simulink model "protocol_nanhang"  (R2023a)
settings: Solver=ode5  StartTime=0.0  StopTime=inf  FixedStep=0.001  RelTol=1e-3
undefined symbols (not defined in the file or in its folder): LF
libraries: instrumentseriallib x6, sldrtlib x1
settings Model: Creator=DELL  LastModifiedBy=DELL
settings HardwareCC: ProdBitPerLong=64  ProdHWDeviceType=Intel->x86-64 (Linux 64)
settings ModelReferenceCC: EnableRefExpFcnMdlSchedulingChecks=on
settings RTWCC: Description=Simulink Desktop Real-Time  SystemTargetFile=sldrt.tlc  TemplateMakefile=sldrt.tmf  RTWCompilerOptimization=on
settings CodeAppCC: MaxIdLength=95
settings SimulinkDesktopRealTimeCC: TargetLibSuffix=_sldrt.a  TargetPreCompLibLocation=C:\Program Files\MATLAB\R2023a\toolbox\sldrt\lib\win64

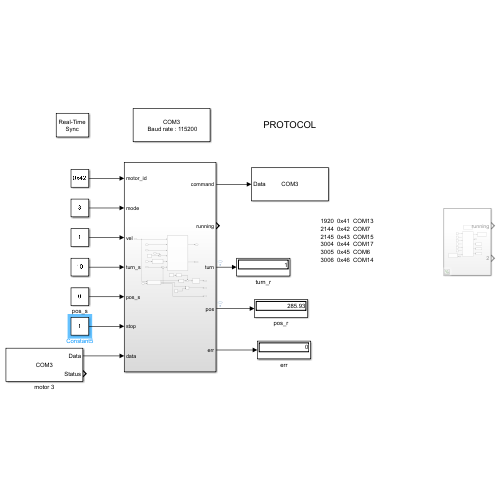
[thumbnail: Simulink's stored preview of the top-level diagram]
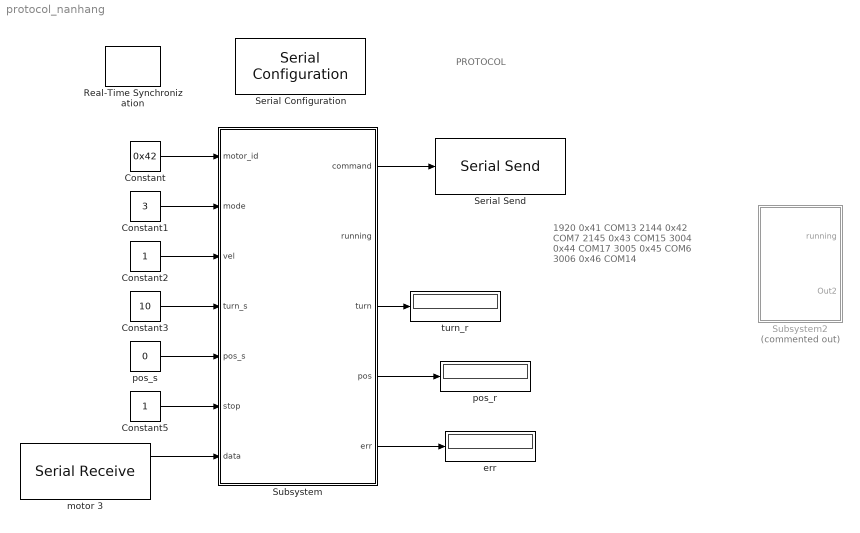
== system protocol_nanhang ==
  note: PROTOCOL
  note: 1920  0x41  COM13
      | 2144  0x42  COM7
      | 2145  0x43  COM15
      | 3004  0x44  COM17
      | 3005  0x45  COM6
      | 3006  0x46  COM14
  Constant : Constant  Value=0x42
  Constant1 : Constant  Value=3
  Constant2 : Constant
  Constant3 : Constant  Value=10
  Constant5 : Constant
  Real-Time Synchronization : sldrtlib/Real-Time Synchronization  SampleTime=0.1  MaxMissedTicks=10  ShowMissedTicks=off  YieldWhenWaiting=off
  Serial Configuration : instrumentseriallib/Serial Configuration  Priority=-200000  PortSel=COM3  Port=COM3  ComPort=COM3  BaudRate=115200  DataBits=8  Parity=none  StopBits=1  ByteOrder=little-endian  FlowControl=none  Timeout=10  SimulateUsing=Interpreted execution  BlockInModel=on  aMode=1
  Serial Send : instrumentseriallib/Serial Send  Priority=1  PortSel=COM3  Port=COM3  ComPort=COM3  Header=[]  Terminator=<none>  CustomTerminator=[]  EnableBlockingMode=off  SimulateUsing=Interpreted execution  BlockInModel=on  aMode=1
  Subsystem : Subsystem
  Subsystem2 : Subsystem  Commented=on
  err : Display
  motor 3 : instrumentseriallib/Serial Receive  Priority=1  PortSel=COM3  Port=COM3  ComPort=COM3  DataType=uint8  SaveDataType=uint8  ToggleHeader=off  Header=[]  ToggleTerminator=on  Terminator=LF ('\n')  CustomTerminator=[]  InputFormat=Column major  ToggleDataSize=on  DataSize=[1 7]  EnableBlockingMode=off  ActionDataUnavailable=Output last received value  ActionWhenDataUnavailable=Output last received value  CustomValue=0  SampleTime=0.01  SimulateUsing=Interpreted execution  BlockInModel=on  aMode=1
  pos_r : Display
  pos_s : Constant  Value=0
  turn_r : Display
  wires:
  Constant/1 -> Subsystem/1(motor_id)
  Constant1/1 -> Subsystem/2(mode)
  Constant2/1 -> Subsystem/3(vel)
  Constant3/1 -> Subsystem/4(turn_s)
  pos_s/1 -> Subsystem/5(pos_s)
  Constant5/1 -> Subsystem/6(stop)
  motor 3/1 -> Subsystem/7(data)
  Subsystem/1(command) -> Serial Send/1
  Subsystem/3(turn) -> turn_r/1
  Subsystem/4(pos) -> pos_r/1
  Subsystem/5(err) -> err/1

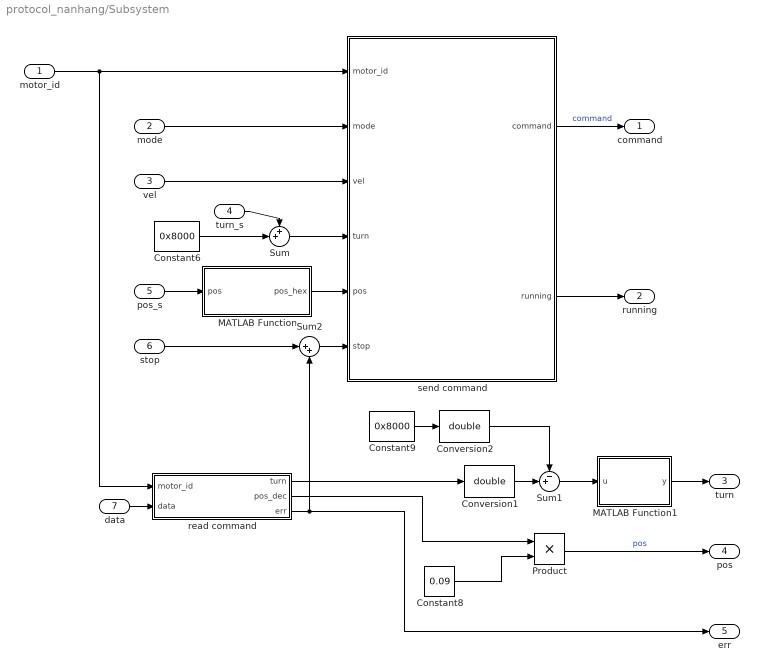
== system protocol_nanhang/Subsystem ==
  motor_id : Inport
  mode : Inport  Port=2
  vel : Inport  Port=3
  turn_s : Inport  Port=4
  pos_s : Inport  Port=5
  stop : Inport  Port=6
  data : Inport  Port=7
  Constant6 : Constant  Value=0x8000
  Constant8 : Constant  Value=0.09
  Constant9 : Constant  Value=0x8000
  Conversion1 : DataTypeConversion  OutDataTypeStr=double  SaturateOnIntegerOverflow=off  RndMeth=Floor
  Conversion2 : DataTypeConversion  OutDataTypeStr=double  SaturateOnIntegerOverflow=off  RndMeth=Floor
  MATLAB Function : MATLAB Function  TreatAsAtomicUnit=on
  MATLAB Function1 : MATLAB Function  TreatAsAtomicUnit=on
  Product : Product
  Sum : Sum  Inputs=++|
  Sum1 : Sum  Inputs=-+|
  Sum2 : Sum  Inputs=|++
  read command : MATLAB Function  TreatAsAtomicUnit=on
  send command : MATLAB Function  TreatAsAtomicUnit=on
  command : Outport
  running : Outport  Port=2
  turn : Outport  Port=3
  pos : Outport  Port=4
  err : Outport  Port=5
  wires:
  Constant6/1 -> Sum/2
  send command/2(running) -> running/1
  MATLAB Function/1(pos_hex) -> send command/5(pos)
  vel/1 -> send command/3(vel)
  read command/2(pos_dec) -> Product/1
  Sum/1 -> send command/4(turn)
  Constant8/1 -> Product/2
  Product/1 -> pos/1  "pos"
  data/1 -> read command/2(data)
  motor_id/1 -> read command/1(motor_id), send command/1(motor_id)
  send command/1(command) -> command/1  "command"
  pos_s/1 -> MATLAB Function/1(pos)
  mode/1 -> send command/2(mode)
  turn_s/1 -> Sum/1
  read command/1(turn) -> Conversion1/1
  Conversion1/1 -> Sum1/2
  Constant9/1 -> Conversion2/1
  Conversion2/1 -> Sum1/1
  Sum1/1 -> MATLAB Function1/1(u)
  MATLAB Function1/1(y) -> turn/1
  read command/3(err) -> err/1, Sum2/2
  stop/1 -> Sum2/1
  Sum2/1 -> send command/6(stop)

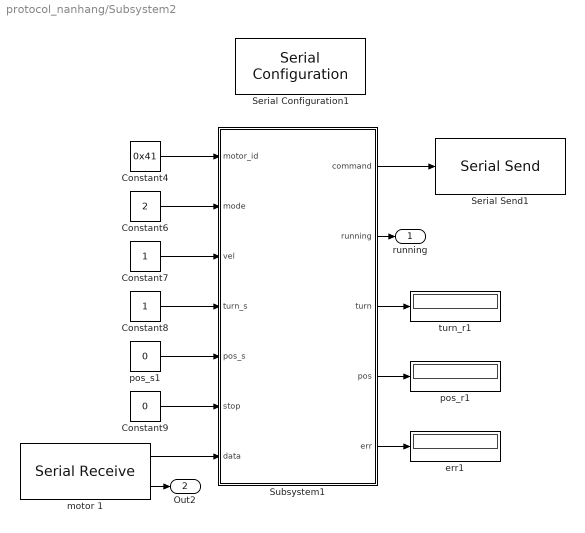
== system protocol_nanhang/Subsystem2 ==
  Constant4 : Constant  Value=0x41
  Constant6 : Constant  Value=2
  Constant7 : Constant
  Constant8 : Constant
  Constant9 : Constant  Value=0
  Serial Configuration1 : instrumentseriallib/Serial Configuration  Priority=-200000  PortSel=COM13  Port=COM13  ComPort=COM13  BaudRate=115200  DataBits=8  Parity=none  StopBits=1  ByteOrder=little-endian  FlowControl=none  Timeout=10  SimulateUsing=Interpreted execution  BlockInModel=on  aMode=1
  Serial Send1 : instrumentseriallib/Serial Send  Priority=1  PortSel=COM13  Port=COM13  ComPort=COM13  Header=[]  Terminator=<none>  CustomTerminator=[]  EnableBlockingMode=off  SimulateUsing=Interpreted execution  BlockInModel=on  aMode=1
  Subsystem1 : Subsystem
  err1 : Display
  motor 1 : instrumentseriallib/Serial Receive  Priority=1  PortSel=COM13  Port=COM13  ComPort=COM13  DataType=uint8  SaveDataType=uint8  ToggleHeader=off  Header=[]  ToggleTerminator=on  Terminator=LF ('\n')  CustomTerminator=[]  InputFormat=Column major  ToggleDataSize=on  DataSize=[1 7]  EnableBlockingMode=off  ActionDataUnavailable=Output last received value  ActionWhenDataUnavailable=Output last received value  CustomValue=0  SampleTime=0.01  SimulateUsing=Interpreted execution  BlockInModel=on  aMode=1
  pos_r1 : Display
  pos_s1 : Constant  Value=0
  turn_r1 : Display
  running : Outport
  Out2 : Outport  Port=2
  wires:
  Constant8/1 -> Subsystem1/4(turn_s)
  Subsystem1/1(command) -> Serial Send1/1
  motor 1/1 -> Subsystem1/7(data)
  Subsystem1/5(err) -> err1/1
  Constant7/1 -> Subsystem1/3(vel)
  Constant6/1 -> Subsystem1/2(mode)
  Subsystem1/4(pos) -> pos_r1/1
  pos_s1/1 -> Subsystem1/5(pos_s)
  Constant4/1 -> Subsystem1/1(motor_id)
  Subsystem1/3(turn) -> turn_r1/1
  Constant9/1 -> Subsystem1/6(stop)
  Subsystem1/2(running) -> running/1
  motor 1/2 -> Out2/1

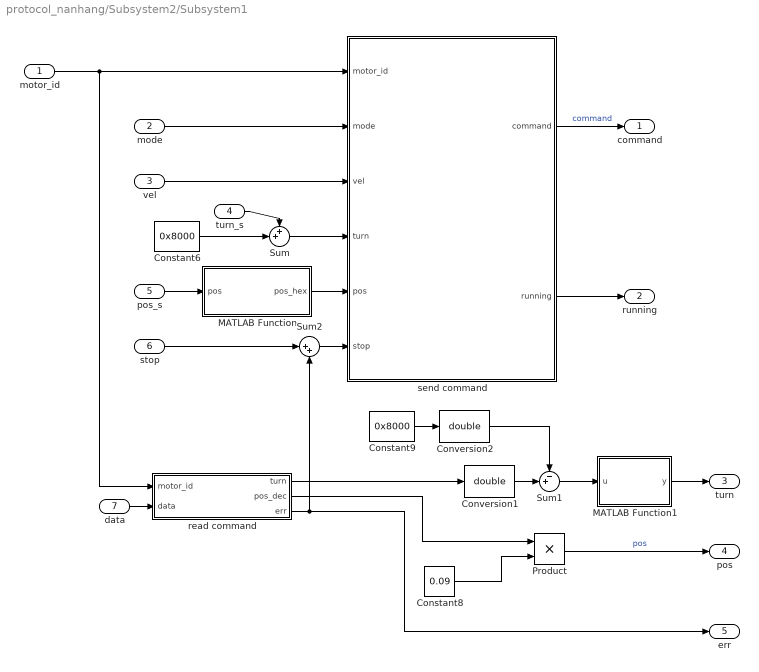
== system protocol_nanhang/Subsystem2/Subsystem1 ==
  motor_id : Inport
  mode : Inport  Port=2
  vel : Inport  Port=3
  turn_s : Inport  Port=4
  pos_s : Inport  Port=5
  stop : Inport  Port=6
  data : Inport  Port=7
  Constant6 : Constant  Value=0x8000
  Constant8 : Constant  Value=0.09
  Constant9 : Constant  Value=0x8000
  Conversion1 : DataTypeConversion  OutDataTypeStr=double  SaturateOnIntegerOverflow=off  RndMeth=Floor
  Conversion2 : DataTypeConversion  OutDataTypeStr=double  SaturateOnIntegerOverflow=off  RndMeth=Floor
  MATLAB Function : MATLAB Function  TreatAsAtomicUnit=on
  MATLAB Function1 : MATLAB Function  TreatAsAtomicUnit=on
  Product : Product
  Sum : Sum  Inputs=++|
  Sum1 : Sum  Inputs=-+|
  Sum2 : Sum  Inputs=|++
  read command : MATLAB Function  TreatAsAtomicUnit=on
  send command : MATLAB Function  TreatAsAtomicUnit=on
  command : Outport
  running : Outport  Port=2
  turn : Outport  Port=3
  pos : Outport  Port=4
  err : Outport  Port=5
  wires:
  Constant6/1 -> Sum/2
  send command/2(running) -> running/1
  MATLAB Function/1(pos_hex) -> send command/5(pos)
  vel/1 -> send command/3(vel)
  read command/2(pos_dec) -> Product/1
  Sum/1 -> send command/4(turn)
  Constant8/1 -> Product/2
  Product/1 -> pos/1  "pos"
  data/1 -> read command/2(data)
  motor_id/1 -> read command/1(motor_id), send command/1(motor_id)
  send command/1(command) -> command/1  "command"
  pos_s/1 -> MATLAB Function/1(pos)
  mode/1 -> send command/2(mode)
  turn_s/1 -> Sum/1
  read command/1(turn) -> Conversion1/1
  Conversion1/1 -> Sum1/2
  Constant9/1 -> Conversion2/1
  Conversion2/1 -> Sum1/1
  Sum1/1 -> MATLAB Function1/1(u)
  MATLAB Function1/1(y) -> turn/1
  read command/3(err) -> err/1, Sum2/2
  stop/1 -> Sum2/1
  Sum2/1 -> send command/6(stop)

== matlab function protocol_nanhang/Subsystem/read command ==
  data: motor_id input; data input; turn output; pos_dec output; err output
function [turn,pos_dec,err] = fcn(motor_id, data)
err=0;
turn=0x8000;
pos_dec=0x0000;
if data(1)~=motor_id
    err=1;
    return
end
if data(2)~=0x54
    err=2;
    return
end
turn = uint16(data(3))*0x100 + uint16(data(4));
pos = uint16(data(5))*0x100 + uint16(data(6));
pos_dec = 0x0000;
mult = 1;
while pos>0
    p1 = mod(pos,0x0010);
    pos = pos - p1;
    pos = pos/0x0010;
    pos_dec = pos_dec + p1*mult;
    mult = mult*10;
end

== matlab function protocol_nanhang/Subsystem/send command ==
  data: motor_id input; mode input; vel input; command output; turn input; running output; pos input; stop input
function [command ,running]= fcn(motor_id, mode, vel,turn,pos,stop)
    command = uint8(zeros(1,16));
    command(9:16) = [motor_id 0x51 0 0 0 0 0 0x0A];

    command(8) = 0x0A;
    command(1) = motor_id;
    running = 1;
    % force stop
    if  stop == 1
        command(2) = 0x53;       
        running = 0;
        return        
    end

    % set mode
    switch mode
        % continues velocity loop
        case 1
            if vel>0
                command(2) = 0x44;
            elseif vel<0
                command(2)=0x55;   
            else
                command(2) = 0x53;
                running = 0;   
            end
            command(7) = abs(vel);
        % impulse velocity loop
        case 2
            if vel>0
                command(2) = 0x46;
            elseif vel<0
                command(2)=0x56;  
            else
                command(2) = 0x53;
                running = 0;                   
            end
            command(7) = abs(vel);
        % coontinue position loop
        case 3
            command(2) = 2;
            command(3) = uint8((turn-mod(turn,0x100))/0x100);
            command(4) = uint8(mod(turn,0x100));
            command(5) = uint8((pos-mod(pos,0x100))/0x100);
            command(6) = uint8(mod(pos,0x100));            
            command(7) = abs(vel);
        % impulse position loop
        case 4
            command(2) = 3;
            command(3) = uint8((turn-mod(turn,0x100))/0x100);
            command(4) = uint8(mod(turn,0x100));
            command(5) = uint8((pos-mod(pos,0x100))/0x100);
            command(6) = uint8(mod(pos,0x100));                
            command(7) = abs(vel);
        case 5
            command(2) = 0x52;
        otherwise
            command(2) = 0x53;       
            running = 0;
    end
end

== matlab function protocol_nanhang/Subsystem/MATLAB Function ==
  data: pos input; pos_hex output
function pos_hex = fcn(pos)
pos = pos/0.09;
pos_hex = 0x0000;
mult = 1;
while pos>0
    digit = mod(pos,10);
    pos = pos - digit;
    pos = pos/10;
    pos_hex = pos_hex + uint16(mult*digit);
    mult = mult*16;
end

== matlab function protocol_nanhang/Subsystem/MATLAB Function1 ==
  data: u input; y output
function y = adjust_init(u)
if(u<=-32767)
    y=0;
else
    y = u;
end

== matlab function protocol_nanhang/Subsystem2/Subsystem1/MATLAB Function ==
  data: pos input; pos_hex output
function pos_hex = fcn(pos)
pos = pos/0.09;
pos_hex = 0x0000;
mult = 1;
while pos>0
    digit = mod(pos,10);
    pos = pos - digit;
    pos = pos/10;
    pos_hex = pos_hex + uint16(mult*digit);
    mult = mult*16;
end

== matlab function protocol_nanhang/Subsystem2/Subsystem1/MATLAB Function1 ==
  data: u input; y output
function y = adjust_init(u)
if(u<=-32767)
    y=0;
else
    y = u;
end

== matlab function protocol_nanhang/Subsystem2/Subsystem1/read command ==
  data: motor_id input; data input; turn output; pos_dec output; err output
function [turn,pos_dec,err] = fcn(motor_id, data)
err=0;
turn=0x8000;
pos_dec=0x0000;
if data(1)~=motor_id
    err=1;
    return
end
if data(2)~=0x54
    err=2;
    return
end
turn = uint16(data(3))*0x100 + uint16(data(4));
pos = uint16(data(5))*0x100 + uint16(data(6));
pos_dec = 0x0000;
mult = 1;
while pos>0
    p1 = mod(pos,0x0010);
    pos = pos - p1;
    pos = pos/0x0010;
    pos_dec = pos_dec + p1*mult;
    mult = mult*10;
end

== matlab function protocol_nanhang/Subsystem2/Subsystem1/send command ==
  data: motor_id input; mode input; vel input; command output; turn input; running output; pos input; stop input
function [command ,running]= fcn(motor_id, mode, vel,turn,pos,stop)
    command = uint8(zeros(1,16));
    command(9:16) = [motor_id 0x51 0 0 0 0 0 0x0A];

    command(8) = 0x0A;
    command(1) = motor_id;
    running = 1;
    % force stop
    if  stop == 1
        command(2) = 0x53;       
        running = 0;
        return        
    end

    % set mode
    switch mode
        % continues velocity loop
        case 1
            if vel>0
                command(2) = 0x44;
            elseif vel<0
                command(2)=0x55;   
            else
                command(2) = 0x53;
                running = 0;   
            end
            command(7) = abs(vel);
        % impulse velocity loop
        case 2
            if vel>0
                command(2) = 0x46;
            elseif vel<0
                command(2)=0x56;  
            else
                command(2) = 0x53;
                running = 0;                   
            end
            command(7) = abs(vel);
        % coontinue position loop
        case 3
            command(2) = 2;
            command(3) = uint8((turn-mod(turn,0x100))/0x100);
            command(4) = uint8(mod(turn,0x100));
            command(5) = uint8((pos-mod(pos,0x100))/0x100);
            command(6) = uint8(mod(pos,0x100));            
            command(7) = abs(vel);
        % impulse position loop
        case 4
            command(2) = 3;
            command(3) = uint8((turn-mod(turn,0x100))/0x100);
            command(4) = uint8(mod(turn,0x100));
            command(5) = uint8((pos-mod(pos,0x100))/0x100);
            command(6) = uint8(mod(pos,0x100));                
            command(7) = abs(vel);
        case 5
            command(2) = 0x52;
        otherwise
            command(2) = 0x53;       
            running = 0;
    end
end
